simulink subsystem "PvtSubSys_VSM_HOD"  (R2020b)
settings: Solver=VariableStepAuto  StartTime=0.0  StopTime=10.0  RelTol=1e-3
values from neighbouring files (symbols this model uses):
  P_VSM_HOD_DrvTrqFlterTIme = 0.5    [HOD.sldd]
  P_VSM_HOD_HandsOff_Tr = 0.23    [HOD.sldd]
  P_VSM_HOD_Handson_TimeInsertPoint : value not decoded    [HOD.sldd]
  P_VSM_HOD_HandsOn_Tr = 0.35    [HOD.sldd]
  P_VSM_HOD_Handson_TrqInsertPoint : value not decoded    [HOD.sldd]
  P_VSM_HOD_HWA_HandsOffLev1TimeCnt = 6000.0    [HOD.sldd]
  P_VSM_HOD_HWA_HandsOffLev2TimeCnt = 6150.0    [HOD.sldd]
  P_VSM_HOD_HWA_HandsOffLev3TimeCnt = 6350.0    [HOD.sldd]
  P_VSM_HOD_HWA_HandsOffLev4TimeCnt = 6600.0    [HOD.sldd]
  P_VSM_HOD_LCKTJA_HandsOffLev1TimeCnt = 6000.0    [HOD.sldd]
  P_VSM_HOD_LCKTJA_HandsOffLev2TimeCnt = 6150.0    [HOD.sldd]
  P_VSM_HOD_LCKTJA_HandsOffLev3TimeCnt = 6350.0    [HOD.sldd]
  P_VSM_HOD_LCKTJA_HandsOffLev4TimeCnt = 6600.0    [HOD.sldd]
libraries: simulink x3, TrueDurationTime x2
settings Model: Creator=GW00133806  LastModifiedBy=GW00201299

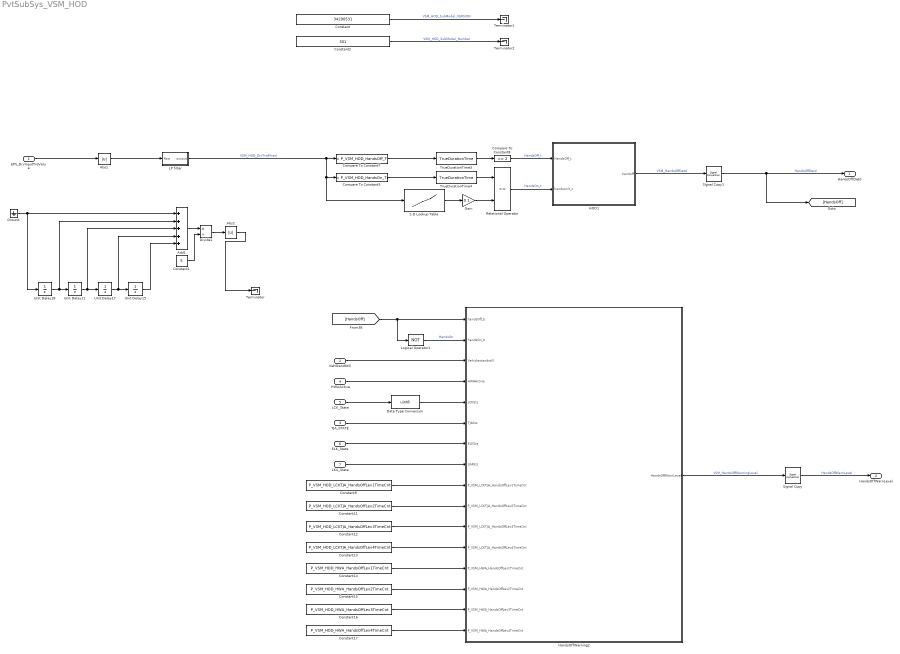
== system PvtSubSys_VSM_HOD ==
  EPS_DrvInputTrqValue : Inport  OutDataTypeStr=single
  VehStandStill : Inport  Port=2  OutDataTypeStr=uint8
  TJA_STATE : Inport  Port=3  OutDataTypeStr=Enum: TJA_STATE
  HWAActive : Inport  Port=4  OutDataTypeStr=boolean
  LCK_State : Inport  Port=5  OutDataTypeStr=Enum: LCK_STATE
  ELK_State : Inport  Port=6  OutDataTypeStr=Enum: ELKSTATE
  LKA_State : Inport  Port=7  OutDataTypeStr=Enum: STATE
  1-D Lookup Table : Lookup_n-D  NumberOfTableDimensions=1  BreakpointsForDimension1=P_VSM_HOD_Handson_TrqInsertPoint  BreakpointsForDimension1DataTypeStr=single  Table=P_VSM_HOD_Handson_TimeInsertPoint  TableDataTypeStr=single  IntermediateResultsDataTypeStr=single  ExtrapMethod=Clip  InternalRulePriority=Speed  OutDataTypeStr=single  RndMeth=Simplest  FractionDataTypeStr=single  InputSameDT=on
  Abs1 : Abs
  Abs2 : Abs
  Add1 : Sum  Inputs=+++++
  Compare To Constant5 : simulink/Logic and Bit Operations/Compare To Constant  relop=>  const=P_VSM_HOD_HandsOn_Tr  OutDataTypeStr=boolean
  Compare To Constant7 : simulink/Logic and Bit Operations/Compare To Constant  relop=<  const=P_VSM_HOD_HandsOff_Tr  OutDataTypeStr=boolean
  Compare To Constant8 : simulink/Logic and Bit Operations/Compare To Constant  relop=>=  const=2  OutDataTypeStr=boolean
  Constant : Constant  Value=34290531  OutDataTypeStr=uint32
  Constant1 : Constant  Value=5
  Constant11 : Constant  Value=P_VSM_HOD_LCKTJA_HandsOffLev2TimeCnt
  Constant12 : Constant  Value=P_VSM_HOD_LCKTJA_HandsOffLev3TimeCnt
  Constant13 : Constant  Value=P_VSM_HOD_LCKTJA_HandsOffLev4TimeCnt
  Constant14 : Constant  Value=P_VSM_HOD_HWA_HandsOffLev1TimeCnt
  Constant15 : Constant  Value=P_VSM_HOD_HWA_HandsOffLev2TimeCnt
  Constant16 : Constant  Value=P_VSM_HOD_HWA_HandsOffLev3TimeCnt
  Constant17 : Constant  Value=P_VSM_HOD_HWA_HandsOffLev4TimeCnt
  Constant2 : Constant  Value=301  OutDataTypeStr=uint16
  Constant9 : Constant  Value=P_VSM_HOD_LCKTJA_HandsOffLev1TimeCnt
  Data Type Conversion : DataTypeConversion  OutDataTypeStr=uint8
  Divide1 : Product  Inputs=*/
  Gain : Gain  Gain=0.1
  Ground : Ground
  HOD1 : Stateflow chart  TreatAsAtomicUnit=on
  HandsOffWarning2 : Stateflow chart  TreatAsAtomicUnit=on
  LP filter : Subsystem
  Logical Operator1 : Logic  Operator=NOT  AllPortsSameDT=off  OutDataTypeStr=boolean
  Relational Operator : RelationalOperator  OutDataTypeStr=boolean  RndMeth=Simplest
  Signal Copy : SignalConversion  OverrideOpt=off
  Signal Copy1 : SignalConversion  OverrideOpt=off
  Terminator : Terminator
  Terminator1 : Terminator
  Terminator2 : Terminator
  TrueDurationTime3 : TrueDurationTime/TrueDurationTime  TCycle=0.02
  TrueDurationTime4 : TrueDurationTime/TrueDurationTime  TCycle=0.02
  Unit Delay{11,15,17..18} (4 alike) : UnitDelay  SampleTime=-1  HasFrameUpgradeWarning=on
  HandsOffDetd : Outport  OutDataTypeStr=boolean
  HandsOffWarnLevel : Outport  Port=2  OutDataTypeStr=uint8
  wires:
  Ground/1 -> Unit Delay18/1, Add1/1
  Gain/1 -> Relational Operator/2
  1-D Lookup Table/1 -> Gain/1
  Constant17/1 -> HandsOffWarning2/16(P_VSM_HWA_HandsOffLev4TimeCnt)
  Constant12/1 -> HandsOffWarning2/11(P_VSM_LCKTJA_HandsOffLev3TimeCnt)
  Constant9/1 -> HandsOffWarning2/9(P_VSM_LCKTJA_HandsOffLev1TimeCnt)
  Constant14/1 -> HandsOffWarning2/13(P_VSM_HWA_HandsOffLev1TimeCnt)
  Constant16/1 -> HandsOffWarning2/15(P_VSM_HWA_HandsOffLev3TimeCnt)
  Constant13/1 -> HandsOffWarning2/12(P_VSM_LCKTJA_HandsOffLev4TimeCnt)
  Constant11/1 -> HandsOffWarning2/10(P_VSM_LCKTJA_HandsOffLev2TimeCnt)
  Constant15/1 -> HandsOffWarning2/14(P_VSM_HWA_HandsOffLev2TimeCnt)
  Logical Operator1/1 -> HandsOffWarning2/2(handsOn_b)  "HandsOn"
  Unit Delay18/1 -> Unit Delay11/1, Add1/2
  HWAActive/1 -> HandsOffWarning2/4(HWAActive)
  ELK_State/1 -> HandsOffWarning2/7(ELKSts)
  Compare To Constant7/1 -> TrueDurationTime3/1
  Compare To Constant5/1 -> TrueDurationTime4/1
  Divide1/1 -> Abs2/1
  Unit Delay17/1 -> Add1/4, Unit Delay15/1
  TJA_STATE/1 -> HandsOffWarning2/6(TJASts)
  TrueDurationTime3/1 -> Compare To Constant8/1
  LP filter/1(output) -> Compare To Constant7/1, Compare To Constant5/1, 1-D Lookup Table/1  "VSM_HOD_DrvTrqFilted"
  TrueDurationTime4/1 -> Relational Operator/1
  Unit Delay15/1 -> Add1/5
  LKA_State/1 -> HandsOffWarning2/8(LKASts)
  Unit Delay11/1 -> Add1/3, Unit Delay17/1
  Add1/1 -> Divide1/1
  Constant1/1 -> Divide1/2
  Signal Copy/1 -> HandsOffWarnLevel/1  "HandsOffWarnLevel"
  EPS_DrvInputTrqValue/1 -> Abs1/1
  LCK_State/1 -> Data Type Conversion/1
  [HandsOff] -> HandsOffWarning2/1(handsOff_b), Logical Operator1/1
  Signal Copy1/1 -> HandsOffDetd/1, [HandsOff]  "HandsOffDetd"
  Relational Operator/1 -> HOD1/2(handson3_t)  "HandsOn_t"
  Compare To Constant8/1 -> HOD1/1(HandsOff_t)  "HandsOff_t"
  HOD1/1(handoff) -> Signal Copy1/1  "VSM_HandsOffDetd"
  HandsOffWarning2/1(HandsOffWarnLevel) -> Signal Copy/1  "VSM_HandsOffWarningLevel"
  VehStandStill/1 -> HandsOffWarning2/3(Vehiclestandstill)
  Abs1/1 -> LP filter/1(Raw)
  Abs2/1 -> Terminator/1
  Constant2/1 -> Terminator2/1  "VSM_HOD_SubModel_Number"
  Constant/1 -> Terminator1/1  "VSM_HOD_SubModel_VERSION"
  Data Type Conversion/1 -> HandsOffWarning2/5(LCKSts)

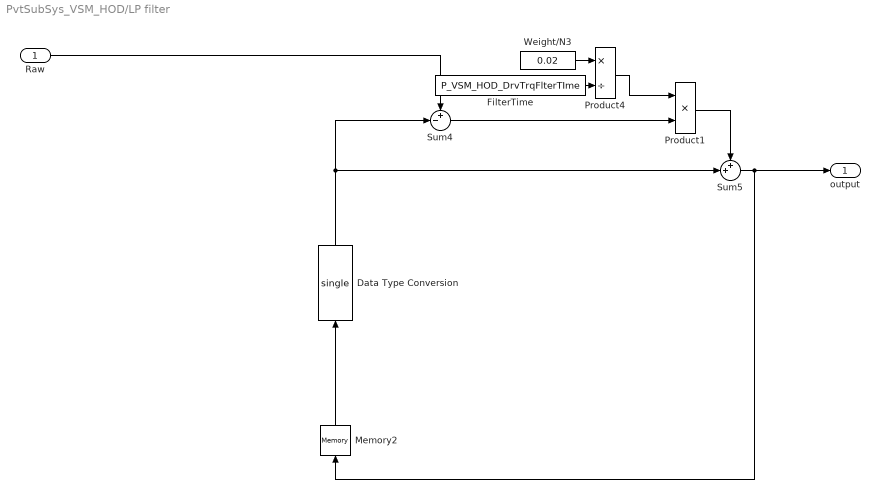
== system PvtSubSys_VSM_HOD/LP filter ==
  Raw : Inport
  Data Type Conversion : DataTypeConversion  OutDataTypeStr=single
  FilterTime : Constant  Value=P_VSM_HOD_DrvTrqFlterTIme  OutDataTypeStr=single
  Memory2 : Memory  InheritSampleTime=on
  Product1 : Product  RndMeth=Zero
  Product4 : Product  Inputs=*/  RndMeth=Zero
  Sum4 : Sum  Inputs=+-|
  Sum5 : Sum  Inputs=++|
  Weight/N3 : Constant  Value=0.02  OutDataTypeStr=single
  output : Outport
  wires:
  Memory2/1 -> Data Type Conversion/1
  Sum4/1 -> Product1/2
  Sum5/1 -> Memory2/1, output/1
  Product1/1 -> Sum5/1
  Raw/1 -> Sum4/1
  Weight/N3/1 -> Product4/1
  Product4/1 -> Product1/1
  FilterTime/1 -> Product4/2
  Data Type Conversion/1 -> Sum4/2, Sum5/2

== stateflow chart PvtSubSys_VSM_HOD/HOD1 ==
  settings: executeAtInitialization=1
  state HandsOn
    en:
    handoff=false;
  state HandsOff
    en:
    handoff=true;
  (default) -> HandsOn
  HandsOn -> HandsOff : [HandsOff_t]
  HandsOff -> HandsOn : [handson3_t]
  data: HandsOff_t input boolean; handoff output boolean; handson3_t input boolean

== stateflow chart PvtSubSys_VSM_HOD/HandsOffWarning2 ==
  settings: executeAtInitialization=1
  state Main [parallel]
    settings: executionOrder=4
    state NoWarning
      en:
      HandsOffWarnLevel=0;
      Cnt_LCK = 0;
      Cnt = 0;
      Cnt2 = 0;
    state WarningLevel1
      en:
      HandsOffWarnLevel=1;
    state WarningLevel2
      en:
      HandsOffWarnLevel=2;
    state WarningLevel3
      en:
      HandsOffWarnLevel=3;
    state WarningLevel4
      en:
      HandsOffWarnLevel=4;
    state WarningLevel5
      en:
      HandsOffWarnLevel=5;
      du:
      Cnt_LCK=min(500,Cnt_LCK+1);
    (default) -> NoWarning
    NoWarning -> WarningLevel1 : [Cnt>P_VSM_LCKTJA_HandsOffLev1TimeCnt||...
        | Cnt2>P_VSM_HWA_HandsOffLev1TimeCnt]
    WarningLevel1 -> NoWarning [order 1] : [HandOn_condition==1]
    WarningLevel2 -> NoWarning [order 2] : [HandOn_condition==1]
    WarningLevel3 -> NoWarning [order 3] : [HandOn_condition==1]
    WarningLevel4 -> NoWarning : [HandOn_condition==1]
    WarningLevel5 -> NoWarning : [handsOn_b||HWAActive==true||...
        | Vehiclestandstill==1||Cnt_LCK>250]
    WarningLevel1 -> WarningLevel2 [order 2] : [Cnt>P_VSM_LCKTJA_HandsOffLev2TimeCnt||...
        | Cnt2>P_VSM_HWA_HandsOffLev2TimeCnt]
    WarningLevel2 -> WarningLevel3 [order 1] : [Cnt>P_VSM_LCKTJA_HandsOffLev3TimeCnt||...
        | Cnt2>P_VSM_HWA_HandsOffLev3TimeCnt]
    WarningLevel3 -> (junction 58) [order 2] : [Cnt>P_VSM_LCKTJA_HandsOffLev4TimeCnt]
    WarningLevel3 -> WarningLevel4 [order 1] : [Cnt2>P_VSM_HWA_HandsOffLev4TimeCnt]
    (junction 58) -> WarningLevel4 [order 2]
    (junction 58) -> WarningLevel5 [order 1] : [(TJASts~=3)&&(TJASts~=6)&&(TJASts~=9)]
  state Time [parallel]
    settings: executionOrder=1
    state HandsOn
      en:
      Cnt=0;
      HandOn_condition = true;
    state HandsOff
      en:
      Cnt=0;
      du:
      Cnt=min(9000,Cnt+1);
      HandOn_condition = false;
    (default) -> HandsOn
    Time.HandsOff -> HandsOn : [~((handsOff_b)&&(HWAActive==false)&&(Vehiclestandstill==0)&&...
        | ((LCKSts==3)||(TJASts==3)||(TJASts==6)||(TJASts==9)))]
    HandsOn -> Time.HandsOff : [(handsOff_b)&&(HWAActive==false)&&(Vehiclestandstill==0)&&...
        | ((LCKSts==3)||(TJASts==3)||(TJASts==6)||(TJASts==9))]
  state Time2 [parallel]
    settings: executionOrder=2
    state HWAHandsOn
      en:
      Cnt2=0;
      HandOn_condition = true;
    state HWAHandsOff
      en:
      Cnt2=0;
      du:
      Cnt2=min(9000,Cnt2+1);
      HandOn_condition = false;
    (default) -> HWAHandsOn
    HWAHandsOff -> HWAHandsOn : [~((handsOff_b)&&(HWAActive==true)&&(Vehiclestandstill==0))]
    HWAHandsOn -> HWAHandsOff : [(handsOff_b)&&(HWAActive==true)&&(Vehiclestandstill==0)]
  state LKA_ELK_HandsOfwarning [parallel]
    du:
    Cnt_Time =Cnt_Time +1;
    if (Cnt_Time>9000)||(~(handsOff_b))
    Cnt_Time=0;
    Cnt_Inter = 0;
    Handsoff_cntK1 = zeros(100,1);
    end
    settings: executionOrder=3
    state Handson_State [parallel]
      settings: executionOrder=2
      state State_Wait
        en:
        Handsoff_cnt = 0;
        HandsOffWarnLevel = 0;
      state HandsOff
        en:
        Hands0ff_Cnt =Cnt_Inter;
        du:
        if Hands0ff_Cnt ~=Cnt_Inter
        Hands0ff_Cnt =Cnt_Inter;
        Handsoff_cnt = 0；
        end
        Handsoff_cnt=Handsoff_cnt+1
        if Cnt_Inter~=1
        HandsOffWarnLevel = 6;
        end
      (default) -> State_Wait
      (junction 297) -> State_Wait
      LKA_ELK_HandsOfwarning.Handson_State.HandsOff -> (junction 297) [order 1] : [(Cnt_Inter>2&&Handsoff_cnt>Handsoff_cntK1(Hands0ff_Cnt-1)+500)&&Warn_State==0||...
          | (Cnt_Inter==2&&Warn_State==0&&Handsoff_cnt>Handsoff_cntK1(Hands0ff_Cnt))]
      State_Wait -> LKA_ELK_HandsOfwarning.Handson_State.HandsOff : [Cnt_Inter>=2&&Warn_State==1]
      LKA_ELK_HandsOfwarning.Handson_State.HandsOff -> State_Wait [order 2] : [handsOn_b||(LKASts==0&&ELKSts==0)||(LCKSts~=0)||(Vehiclestandstill~=0)]
    state LKAELK_State [parallel]
      settings: executionOrder=1
      state Nowarning
        en:
        Warn_State=0;
        Cnt_Inter_Time =0;
      state InterveneWaiting
        en:
        Cnt_Inter = 0;
      state Warning
        en:
        Cnt_Inter_Time = 0;
        Warn_State=1;
        Inter_Flag=false;
        du:
        Cnt_Inter_Time=min(Cnt_Inter_Time+1, 15000);
        if handsOff_b && Inter_Flag~=true
        Cnt_Inter = Cnt_Inter+1;
        Inter_Flag=true;
        end
      (default) -> InterveneWaiting
      Nowarning -> InterveneWaiting [order 1] : [~((HWAActive==false)&&(Vehiclestandstill==0)&&(LCKSts~=3)&&...
          | (TJASts~=3)&&(TJASts~=6)&&(TJASts~=9))]
      Nowarning -> (junction 240) [order 2]
      Warning -> InterveneWaiting [order 1] : [~((HWAActive==false)&&(Vehiclestandstill==0)&&(LCKSts~=3)&&...
          | (TJASts~=3)&&(TJASts~=6)&&(TJASts~=9))]
          | {Handsoff_cntK1(Cnt_Inter)=Cnt_Inter_Time;}
      InterveneWaiting -> Warning : [(HWAActive==false)&&(Vehiclestandstill==0)&&(LCKSts~=3)&&...
          | ((TJASts~=3)&&(TJASts~=6)&&(TJASts~=9))&&((LKASts==4)||(LKASts==5)||...
          | ((ELKSts~=0)&&(ELKSts~=1)&&(ELKSts~=2)&&(ELKSts~=9)))]{Cnt_Time =0;}
      (junction 240) -> Warning : [(HWAActive==false)&&(Vehiclestandstill==0)&&(LCKSts~=3)&&...
          | ((TJASts~=3)&&(TJASts~=6)&&(TJASts~=9))&&((LKASts==4)||(LKASts==5)||...
          | ((ELKSts~=0)&&(ELKSts~=1)&&(ELKSts~=2)&&(ELKSts~=9)))]
      Warning -> Nowarning [order 2] : [LKASts~=4&&LKASts~=5&&...
          | (ELKSts==0||ELKSts==1||ELKSts==2||ELKSts==9)]
          | {Handsoff_cntK1(Cnt_Inter)=Cnt_Inter_Time;}
  data: Cnt local double; handsOff_b input boolean; handsOn_b input boolean; Vehiclestandstill input uint8; HandsOffWarnLevel output uint8; HWAActive input boolean; LCKSts input uint8; TJASts input Enum: TJA_STATE; Cnt2 local double; ELKSts input Enum: ELKSTATE; LKASts input Enum: STATE; HandOn_condition local boolean; Cnt_Inter local double; Cnt_Time local double =0; Handsoff_cnt local double; Handsoff_cntK1 local double size=[100,1] =zeros(100,0); Cnt_LCK local =0; P_VSM_LCKTJA_HandsOffLev1TimeCnt input single; P_VSM_LCKTJA_HandsOffLev2TimeCnt input single; P_VSM_LCKTJA_HandsOffLev3TimeCnt input single; P_VSM_LCKTJA_HandsOffLev4TimeCnt input single; P_VSM_HWA_HandsOffLev1TimeCnt input single; P_VSM_HWA_HandsOffLev2TimeCnt input single; P_VSM_HWA_HandsOffLev3TimeCnt input single; P_VSM_HWA_HandsOffLev4TimeCnt input single; Cnt_InterK1 local; Cnt_Inter_TimeK1 local =0; Warn_State local =0; Hands0ff_Cnt local; Cnt_Inter_Time local; Inter_Flag local
